simulink subsystem "Subsystem_EncoderDistancia"  (R2023b)
settings: Solver=VariableStepAuto  StartTime=0.0  StopTime=10.0  RelTol=1e-3
libraries: arduinosensorlib x2
settings Model: Creator=Alberto  LastModifiedBy=Alberto

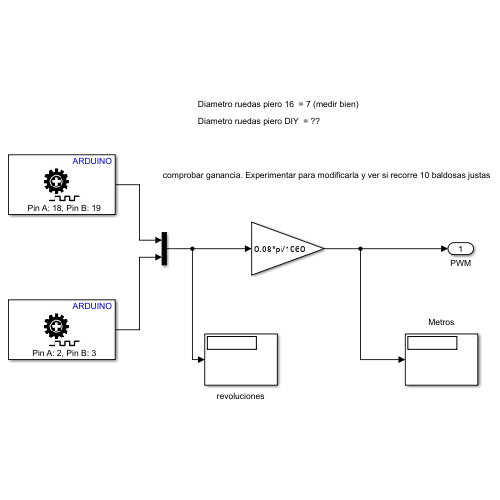
[thumbnail: Simulink's stored preview of the top-level diagram]
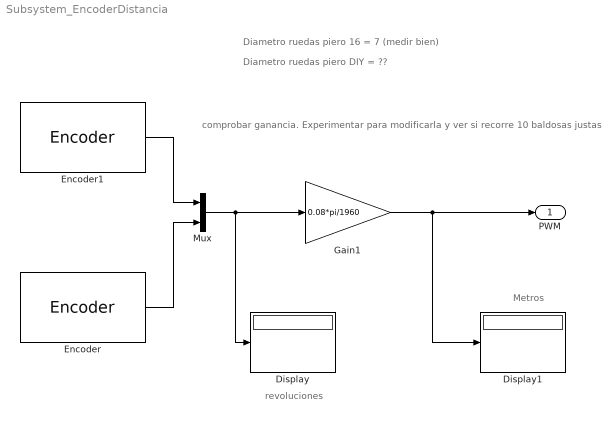
== system Subsystem_EncoderDistancia ==
  note: revoluciones
  note: Metros
  note: comprobar ganancia. Experimentar para modificarla y ver si recorre 10 baldosas justas
  note: Diametro ruedas piero 16 = 7 (medir bien)
  note: Diametro ruedas piero DIY = ??
  Display : Display
  Display1 : Display
  Encoder : arduinosensorlib/Encoder  InputA=2  InputB=3  Mode=No reset  SampleTime=-1
  Encoder1 : arduinosensorlib/Encoder  InputA=18  InputB=19  Mode=No reset  SampleTime=-1
  Gain1 : Gain  Gain=0.08*pi/1960
  Mux : Mux  Inputs=2
  PWM : Outport
  wires:
  Mux/1 -> Gain1/1, Display/1
  Gain1/1 -> PWM/1, Display1/1
  Encoder1/1 -> Mux/1
  Encoder/1 -> Mux/2
